simulink model "Fig2"  (R2015a)
settings: Solver=ode45  StartTime=0.0  StopTime=10.0  RelTol=1e-3
libraries: dspvision x1, dspsnks4 x1
settings Model: Creator=Meghna  LastModifiedBy=Meghna

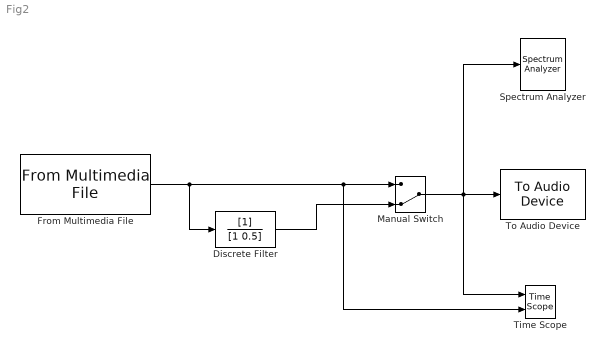
== system Fig2 ==
  Discrete Filter : DiscreteFilter
  From Multimedia File : dspvision/From Multimedia File  inputFilename=speech_dft.mp3  loop=on  numPlays=inf  outputStreams=Audio only  videoDataType=single  audioDataType=double  inheritSampleTime=on  userDefinedSampleTime=1/30  noAudioOutput=off  isIntensityVideo=off  fourcc=RGB  colorVideoFormat=Separate color signals  outputEOF=off  dataOrg=Column-major  audioFrameSize=1024  computeAudioFrameSize=off  outSamplingMode=Sample based
  Manual Switch : ManualSwitch  CurrentSetting=0
  Spectrum Analyzer : SpectrumAnalyzer
  Time Scope : TimeScope  DefaultConfigurationName=spbscopes.TimeScopeBlockCfg  NumInputPorts=2
  To Audio Device : dspsnks4/To Audio Device  deviceName=Default  inheritSampleRate=on  sampleRate=44100  deviceDatatype=Determine from input data type  autoBufferSize=on  bufferSize=4096  queueDuration=1.0  defaultOutputChannelMapping=on  outputChannelMapping=1:2  outputNumUnderrunSamples=off
  wires:
  From Multimedia File/1 -> Discrete Filter/1, Time Scope/2, Manual Switch/1
  Discrete Filter/1 -> Manual Switch/2
  Manual Switch/1 -> Time Scope/1, To Audio Device/1, Spectrum Analyzer/1
